simulink model "topology_comparison_eff"  (R2024b)
settings: Solver=ode23tb  StartTime=0.0  StopTime=4  MaxStep=1e-4  MinStep=1e-9  RelTol=1e-3
InitFcn:
  | sw_freq=60e3;
  | eff_rms_freq=sw_freq/10;
  | V_high=80;
  | 
  | L_ind=300e-6;
  | L_res=20e-3;
  | 
  | MOS_Ron=10e-3;
  | MOS_Vfw=1.2;
  | 
  | DIO_Vfw=0.9;
  | DIO_Ron=2e-3;
  | 
  | TRC_Res=5e-3;
  | 
  | sync_mode=1;
  | 
  | buck_p=0.02;
  | buck_i=0.8;
  | 
  | inter_bdc_p=0.02;
  | inter_bdc_i=0.9;
  | 
  | asym_bdc_p=0.02;
  | asym_bdc_i=1.1;
values from neighbouring files (symbols this model uses):
  runtime = 4    [compare_conv_eff.m]
  timestep = runtime/size(curr_range,2)    [compare_conv_eff.m]
undefined symbols (not defined in the file or in its folder): V_low
libraries: spsMeanLib x14, spsGroundLib x14, spsSeriesRLCBranchLib x14, spsMosfetLib x10, slpidlib x7, spsDCVoltageSourceLib x6, spsMultimeterLib x3, spsDiodeLib x2, embmathops x1, spsStairGeneratorLib x1, spspowerguiLib x1
(part 2 of 2)

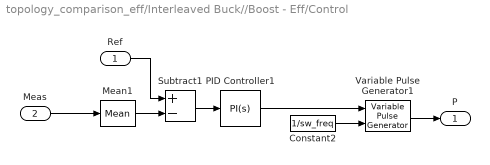
== system topology_comparison_eff/Interleaved Buck//Boost - Eff/Control ==
  Ref : Inport
  Meas : Inport  Port=2
  Constant2 : Constant  Value=1/sw_freq
  Mean1 : spsMeanLib/Mean  Freq=sw_freq/6  Vinit=0  Ts=0
  PID Controller1 : slpidlib/PID Controller  Controller=PI  Form=Parallel  TimeDomain=Continuous-time  UseExternalTs=off  SampleTime=-1  IntegratorMethod=Forward Euler  FilterMethod=Forward Euler  ControllerParametersSource=internal  P=inter_bdc_p  I=inter_bdc_i  UseKiTs=on  D=0  UseExternalDerivativeSource=off  N=100  UseFilter=on  TunerSelectOption=Transfer Function Based (PID Tuner App)  InitialConditionSource=internal  InitialConditionForIntegrator=0.14  InitialConditionForFilter=0  DifferentiatorICPrevScaledInput=0  ExternalReset=none  TrackingMode=off  Kt=1  LimitOutput=on  SatLimitsSource=internal  UpperSaturationLimit=1  LowerSaturationLimit=0.01  LinearizeAsGain=on  AntiWindupMode=none  Kb=1  LimitIntegrator=off  UpperIntegratorSaturationLimit=inf  LowerIntegratorSaturationLimit=-inf  POutMin=[]  POutMax=[]  IOutMin=[]  IOutMax=[]  DOutMin=[]  DOutMax=[]  NOutMin=[]  NOutMax=[]  SumOutMin=[]  SumOutMax=[]  SaturationOutMin=[]  SaturationOutMax=[]  PParamMin=[]  PParamMax=[]  IParamMin=[]  IParamMax=[]  DParamMin=[]  DParamMax=[]  NParamMin=[]  NParamMax=[]  KbParamMin=[]  KbParamMax=[]  KtParamMin=[]  KtParamMax=[]  KbOutMin=[]  KbOutMax=[]  KtOutMin=[]  KtOutMax=[]  IntegratorOutMin=[]  IntegratorOutMax=[]  FilterOutMin=[]  FilterOutMax=[]  SumI1OutMin=[]  SumI1OutMax=[]  SumI2OutMin=[]  SumI2OutMax=[]  SumI3OutMin=[]  SumI3OutMax=[]  SumI4OutMin=[]  SumI4OutMax=[]  SumDOutMin=[]  SumDOutMax=[]  DifferentiatorOutMin=[]  DifferentiatorOutMax=[]  FilterDiffOutCoefMin=[]  FilterDiffOutCoefMax=[]  ReciprocalOutMin=[]  ReciprocalOutMax=[]  SumDenOutMin=[]  SumDenOutMax=[]  SumNumOutMin=[]  SumNumOutMax=[]  DivideOutMin=[]  DivideOutMax=[]  UdiffTsProdOutMin=[]  UdiffTsProdOutMax=[]  NTsProdOutMin=[]  NTsProdOutMax=[]  UintegralTsProdOutMin=[]  UintegralTsProdOutMax=[]  UngainTsProdOutMin=[]  UngainTsProdOutMax=[]  ClampingZeroOutDataTypeStr=Inherit: Inherit via back propagation  ClampingZeroOutMin=[]  ClampingZeroOutMax=[]  FilterDenConstantOutDataTypeStr=Inherit: Inherit via back propagation  FilterDenConstantOutMin=[]  FilterDenConstantOutMax=[]  PCopyOutDataTypeStr=Inherit: Inherit via back propagation  PCopyOutMin=[]  PCopyOutMax=[]  NCopyOutDataTypeStr=Inherit: Inherit via back propagation  NCopyOutMin=[]  NCopyOutMax=[]  IntegratorContinuousStateAttributes=''  IntegratorStateMustResolveToSignalObject=off  IntegratorRTWStateStorageClass=Auto  FilterContinuousStateAttributes=''  FilterStateMustResolveToSignalObject=off  FilterRTWStateStorageClass=Auto  ParallelPVariant=InternalParameters  IdealPVariant=Disabled  IVariant=InternalParameters  DVariant=Disabled  IntegratorVariant=Continuous  SatVariant=Enabled  AWVariant=Passthrough  PCopyVariant=Disabled  TRVariant=Disabled  FdbkBlocksVariant=Forward  IdealPFdbkVariant=Disabled  SatFdbkVariant=Disabled  DerivativeFilterVariant=Disabled  NVariant=Disabled  NCopyVariant=Disabled_SignalSpec  FilterICVariant=Disabled  IntegratorICVariant=InternalICs  ExternalResetVariant=Disabled  TRSumVariant=Passthrough  SumFdbkVariant=Disabled  SumVariant=Sum_PI  TsampFilterVariant=InternalTs  TsampNgainVariant=Passthrough  TsampIntegralVariant=Disabled_SignalSpec  ExternalSaturationOutDataTypeStr=Inherit: Same as second input  DerivativeSourceVariant=Disabled  PreIntVariant=InternalPreInt
  Subtract1 : Sum  Inputs=+-
  Variable Pulse Generator1 : VariablePulseGenerator  AllowZeroPulseWidth=on  SampleTime=0.1
  P : Outport
  wires:
  Meas/1 -> Mean1/1
  PID Controller1/1 -> Variable Pulse Generator1/1
  Constant2/1 -> Variable Pulse Generator1/2
  Mean1/1 -> Subtract1/2
  Subtract1/1 -> PID Controller1/1
  Variable Pulse Generator1/1 -> P/1
  Ref/1 -> Subtract1/1

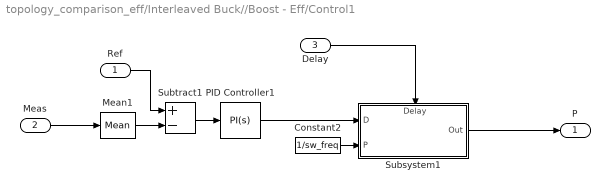
== system topology_comparison_eff/Interleaved Buck//Boost - Eff/Control1 ==
  Ref : Inport
  Meas : Inport  Port=2
  Delay : Inport  Port=3
  Constant2 : Constant  Value=1/sw_freq
  Mean1 : spsMeanLib/Mean  Freq=sw_freq/6  Vinit=0  Ts=0
  PID Controller1 : slpidlib/PID Controller  Controller=PI  Form=Parallel  TimeDomain=Continuous-time  UseExternalTs=off  SampleTime=-1  IntegratorMethod=Forward Euler  FilterMethod=Forward Euler  ControllerParametersSource=internal  P=inter_bdc_p  I=inter_bdc_i  UseKiTs=on  D=0  UseExternalDerivativeSource=off  N=100  UseFilter=on  TunerSelectOption=Transfer Function Based (PID Tuner App)  InitialConditionSource=internal  InitialConditionForIntegrator=0.14  InitialConditionForFilter=0  DifferentiatorICPrevScaledInput=0  ExternalReset=none  TrackingMode=off  Kt=1  LimitOutput=on  SatLimitsSource=internal  UpperSaturationLimit=1  LowerSaturationLimit=0.01  LinearizeAsGain=on  AntiWindupMode=none  Kb=1  LimitIntegrator=off  UpperIntegratorSaturationLimit=inf  LowerIntegratorSaturationLimit=-inf  POutMin=[]  POutMax=[]  IOutMin=[]  IOutMax=[]  DOutMin=[]  DOutMax=[]  NOutMin=[]  NOutMax=[]  SumOutMin=[]  SumOutMax=[]  SaturationOutMin=[]  SaturationOutMax=[]  PParamMin=[]  PParamMax=[]  IParamMin=[]  IParamMax=[]  DParamMin=[]  DParamMax=[]  NParamMin=[]  NParamMax=[]  KbParamMin=[]  KbParamMax=[]  KtParamMin=[]  KtParamMax=[]  KbOutMin=[]  KbOutMax=[]  KtOutMin=[]  KtOutMax=[]  IntegratorOutMin=[]  IntegratorOutMax=[]  FilterOutMin=[]  FilterOutMax=[]  SumI1OutMin=[]  SumI1OutMax=[]  SumI2OutMin=[]  SumI2OutMax=[]  SumI3OutMin=[]  SumI3OutMax=[]  SumI4OutMin=[]  SumI4OutMax=[]  SumDOutMin=[]  SumDOutMax=[]  DifferentiatorOutMin=[]  DifferentiatorOutMax=[]  FilterDiffOutCoefMin=[]  FilterDiffOutCoefMax=[]  ReciprocalOutMin=[]  ReciprocalOutMax=[]  SumDenOutMin=[]  SumDenOutMax=[]  SumNumOutMin=[]  SumNumOutMax=[]  DivideOutMin=[]  DivideOutMax=[]  UdiffTsProdOutMin=[]  UdiffTsProdOutMax=[]  NTsProdOutMin=[]  NTsProdOutMax=[]  UintegralTsProdOutMin=[]  UintegralTsProdOutMax=[]  UngainTsProdOutMin=[]  UngainTsProdOutMax=[]  ClampingZeroOutDataTypeStr=Inherit: Inherit via back propagation  ClampingZeroOutMin=[]  ClampingZeroOutMax=[]  FilterDenConstantOutDataTypeStr=Inherit: Inherit via back propagation  FilterDenConstantOutMin=[]  FilterDenConstantOutMax=[]  PCopyOutDataTypeStr=Inherit: Inherit via back propagation  PCopyOutMin=[]  PCopyOutMax=[]  NCopyOutDataTypeStr=Inherit: Inherit via back propagation  NCopyOutMin=[]  NCopyOutMax=[]  IntegratorContinuousStateAttributes=''  IntegratorStateMustResolveToSignalObject=off  IntegratorRTWStateStorageClass=Auto  FilterContinuousStateAttributes=''  FilterStateMustResolveToSignalObject=off  FilterRTWStateStorageClass=Auto  ParallelPVariant=InternalParameters  IdealPVariant=Disabled  IVariant=InternalParameters  DVariant=Disabled  IntegratorVariant=Continuous  SatVariant=Enabled  AWVariant=Passthrough  PCopyVariant=Disabled  TRVariant=Disabled  FdbkBlocksVariant=Forward  IdealPFdbkVariant=Disabled  SatFdbkVariant=Disabled  DerivativeFilterVariant=Disabled  NVariant=Disabled  NCopyVariant=Disabled_SignalSpec  FilterICVariant=Disabled  IntegratorICVariant=InternalICs  ExternalResetVariant=Disabled  TRSumVariant=Passthrough  SumFdbkVariant=Disabled  SumVariant=Sum_PI  TsampFilterVariant=InternalTs  TsampNgainVariant=Passthrough  TsampIntegralVariant=Disabled_SignalSpec  ExternalSaturationOutDataTypeStr=Inherit: Same as second input  DerivativeSourceVariant=Disabled  PreIntVariant=InternalPreInt
  Subsystem1 : Subsystem
      settings: PortSchema="{\"entries\":[{\"content\":{\"sides\":[{\"content\":{\"connectorIds\":[\"In1\",\"In2\"]},\"type\":\"ConnectorPlacement.EquallySpacedRectSide\",\"uuid\":\"51b045c8-d819-4b7c-a29d-1a54f5fd995d\"},{\"content\":{\"connectorIds\":[\"Out1\"],\"side\":\"RIGHT\"},\"type\":\"ConnectorPlacement.EquallySpacedRectSide\",\"uuid\":\"9f0647dc-9c35-4883-9e64-6da00897cce8\"},{\"content\":{\"connectorIds\":[\"In3\"],\"side\":\"TOP\"},\"type\":\"ConnectorPlacement.EquallySpacedRectSide\",\"uuid\":\"a4aa7abf-9a58-441d-bef7-3a2aafbde944\"}]},\"type\":\"ConnectorPlacement.EquallySpacedConnector\",\"uuid\":\"237ebc79-3794-4318-8db8-2d16dc313947\"}],\"packageUris\":[\"http://schema.mathworks.com/mf0/Connector/R2020b\"],\"version\":\"1.0\"}"
  Subtract1 : Sum  Inputs=+-
  P : Outport
  wires:
  Meas/1 -> Mean1/1
  PID Controller1/1 -> Subsystem1/1(D)
  Mean1/1 -> Subtract1/2
  Subtract1/1 -> PID Controller1/1
  Subsystem1/1(Out) -> P/1
  Ref/1 -> Subtract1/1
  Constant2/1 -> Subsystem1/2(P)
  Delay/1 -> Subsystem1/3(Delay)

== system topology_comparison_eff/Asymetrical Buck//Boost - Eff/Control3/Subsystem3 ==
  D : Inport
  P : Inport  Port=2
  Delay : Inport  Port=3
  Clock1 : Clock
  GreaterThan : RelationalOperator  Operator=>  OutDataTypeStr=boolean  RndMeth=Simplest  InputSameDT=off
  Subsystem : Subsystem
  Out : Outport
  wires:
  Clock1/1 -> GreaterThan/1
  P/1 -> Subsystem/2(P)
  GreaterThan/1 -> Subsystem/Enable
  D/1 -> Subsystem/1(D)
  Delay/1 -> GreaterThan/2
  Subsystem/1(Out) -> Out/1

== system topology_comparison_eff/Asymetrical Buck//Boost - Eff/Control4/Subsystem3 ==
  D : Inport
  P : Inport  Port=2
  Delay : Inport  Port=3
  Clock1 : Clock
  GreaterThan : RelationalOperator  Operator=>  OutDataTypeStr=boolean  RndMeth=Simplest  InputSameDT=off
  Subsystem : Subsystem
  Out : Outport
  wires:
  Clock1/1 -> GreaterThan/1
  P/1 -> Subsystem/2(P)
  GreaterThan/1 -> Subsystem/Enable
  D/1 -> Subsystem/1(D)
  Delay/1 -> GreaterThan/2
  Subsystem/1(Out) -> Out/1

== system topology_comparison_eff/Interleaved Buck//Boost - Eff/Control1/Subsystem1 ==
  D : Inport
  P : Inport  Port=2
  Delay : Inport  Port=3
  Clock1 : Clock
  GreaterThan : RelationalOperator  Operator=>  OutDataTypeStr=boolean  RndMeth=Simplest  InputSameDT=off
  Subsystem : Subsystem
  Out : Outport
  wires:
  Clock1/1 -> GreaterThan/1
  P/1 -> Subsystem/2(P)
  GreaterThan/1 -> Subsystem/Enable
  D/1 -> Subsystem/1(D)
  Delay/1 -> GreaterThan/2
  Subsystem/1(Out) -> Out/1

== system topology_comparison_eff/Asymetrical Buck//Boost - Eff/Control3/Subsystem3/Subsystem ==
  D : Inport
  P : Inport  Port=2
  Enable : EnablePort
  Variable Pulse Generator1 : VariablePulseGenerator  AllowZeroPulseWidth=on  SampleTime=0.1
  Out : Outport
  wires:
  D/1 -> Variable Pulse Generator1/1
  Variable Pulse Generator1/1 -> Out/1
  P/1 -> Variable Pulse Generator1/2

== system topology_comparison_eff/Asymetrical Buck//Boost - Eff/Control4/Subsystem3/Subsystem ==
  D : Inport
  P : Inport  Port=2
  Enable : EnablePort
  Variable Pulse Generator1 : VariablePulseGenerator  AllowZeroPulseWidth=on  SampleTime=0.1
  Out : Outport
  wires:
  D/1 -> Variable Pulse Generator1/1
  Variable Pulse Generator1/1 -> Out/1
  P/1 -> Variable Pulse Generator1/2

== system topology_comparison_eff/Interleaved Buck//Boost - Eff/Control1/Subsystem1/Subsystem ==
  D : Inport
  P : Inport  Port=2
  Enable : EnablePort
  Variable Pulse Generator1 : VariablePulseGenerator  AllowZeroPulseWidth=on  SampleTime=0.1
  Out : Outport
  wires:
  D/1 -> Variable Pulse Generator1/1
  Variable Pulse Generator1/1 -> Out/1
  P/1 -> Variable Pulse Generator1/2
